simulink model "1DoF_controller_example"  (R2024b)
settings: Solver=FixedStepAuto  StartTime=0.0  StopTime=inf  RelTol=1e-3  EnableMultiTasking=on
undefined symbols (not defined in the file): dspblkCoreblockFVToolHelper, gcbh
libraries: px4Peripheralslib x1, slpidlib x1, px4uORBlib x1, sharedtransform x1, simulink_extras x1
settings Model: SimulationMode=external  ExtModeTrigDuration=10  Creator=luker  LastModifiedBy=luker
settings SolverCC: PositivePriorityOrder=on
settings OptimizationCC: EnhancedBackFolding=on  PassReuseOutputArgsAs=Individual arguments  ZeroExternalMemoryAtStartup=off  ZeroInternalMemoryAtStartup=off  MaxStackSize=64  OptimizeBlockOrder=speed  DifferentSizesBufferReuse=on  EfficientTunableParamExpr=on
settings DebuggingCC: ParameterTunabilityLossMsg=error
settings HardwareCC: ProdBitPerPointer=32  ProdBitPerSizeT=32  ProdBitPerPtrDiffT=32  ProdLargestAtomicInteger=Long  ProdLargestAtomicFloat=Double  ProdWordSize=32  ProdLongLongMode=on  ProdHWDeviceType=ARM Compatible->ARM Cortex
settings SFSimCC: MATLABDynamicMemAlloc=off  SimTargetLang=C++
settings RTWCC: Description=Embedded Coder  SystemTargetFile=ert.tlc  HardwareBoard=PX4 Pixhawk Series  TLCOptions="-aInlineSetEventsForThisBaseRateFcn=TLC_FALSE -aSuppressMultiTaskScheduler=TLC_FALSE  -aRateBasedStepFcn=0"  TemplateMakefile=ert_default_tmf  Toolchain=GNU Tools for PX4 Autopilots  TargetLang=C++
settings CodeAppCC: ForceParamTrailComments=on  IgnoreCustomStorageClasses=off  OperatorAnnotations=on  SimulinkDataObjDesc=on  SFDataObjDesc=on  InsertBlockDesc=on
settings ERTTargetCC: ExtModeTransport=3  ExtModeStaticAlloc=on  ExtModeStaticAllocSize=1024  ExtModeMexFile=ext_xcp  ExtModeIntrfLevel=Level2 - Open  InlinedParameterPlacement=Hierarchical

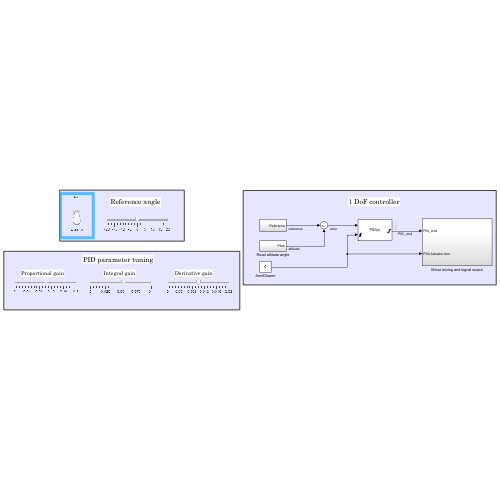
[thumbnail: Simulink's stored preview of the top-level diagram]
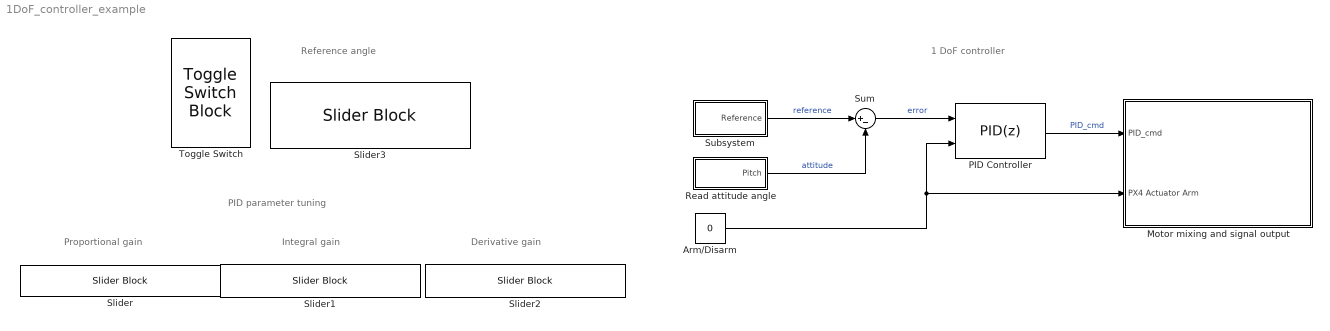
== system 1DoF_controller_example ==
  note: Proportional gain
  note: Reference angle
  note: PID parameter tuning
  note: Integral gain
  note: Derivative gain
  note: 1 DoF controller
  Arm/Disarm : Constant  Value=0
  Motor mixing and signal output : Subsystem
  PID Controller : slpidlib/PID Controller  Controller=PID  Form=Parallel  TimeDomain=Discrete-time  UseExternalTs=off  SampleTime=0.007  IntegratorMethod=Forward Euler  FilterMethod=Forward Euler  ControllerParametersSource=internal  P=0.1027863777089783  I=0.05424823410696267  UseKiTs=off  D=0.01003095975232198  UseExternalDerivativeSource=off  N=60  UseFilter=on  TunerSelectOption=Transfer Function Based (PID Tuner App)  InitialConditionSource=internal  InitialConditionForIntegrator=0  InitialConditionForFilter=0  DifferentiatorICPrevScaledInput=0  ExternalReset=rising  TrackingMode=off  Kt=1  LimitOutput=on  SatLimitsSource=internal  UpperSaturationLimit=0.5  LowerSaturationLimit=-0.5  LinearizeAsGain=off  AntiWindupMode=back-calculation  Kb=100  LimitIntegrator=on  UpperIntegratorSaturationLimit=0.08  LowerIntegratorSaturationLimit=-0.08  POutMin=[]  POutMax=[]  IOutMin=[]  IOutMax=[]  DOutMin=[]  DOutMax=[]  NOutMin=[]  NOutMax=[]  SumOutMin=[]  SumOutMax=[]  SaturationOutMin=[]  SaturationOutMax=[]  PParamMin=[]  PParamMax=[]  IParamMin=[]  IParamMax=[]  DParamMin=[]  DParamMax=[]  NParamMin=[]  NParamMax=[]  KbParamMin=[]  KbParamMax=[]  KtParamMin=[]  KtParamMax=[]  KbOutMin=[]  KbOutMax=[]  KtOutMin=[]  KtOutMax=[]  IntegratorOutMin=[]  IntegratorOutMax=[]  FilterOutMin=[]  FilterOutMax=[]  SumI1OutMin=[]  SumI1OutMax=[]  SumI2OutMin=[]  SumI2OutMax=[]  SumI3OutMin=[]  SumI3OutMax=[]  SumI4OutMin=[]  SumI4OutMax=[]  SumDOutMin=[]  SumDOutMax=[]  DifferentiatorOutMin=[]  DifferentiatorOutMax=[]  FilterDiffOutCoefMin=[]  FilterDiffOutCoefMax=[]  ReciprocalOutMin=[]  ReciprocalOutMax=[]  SumDenOutMin=[]  SumDenOutMax=[]  SumNumOutMin=[]  SumNumOutMax=[]  DivideOutMin=[]  DivideOutMax=[]  UdiffTsProdOutMin=[]  UdiffTsProdOutMax=[]  NTsProdOutMin=[]  NTsProdOutMax=[]  UintegralTsProdOutMin=[]  UintegralTsProdOutMax=[]  UngainTsProdOutMin=[]  UngainTsProdOutMax=[]  ClampingZeroOutDataTypeStr=Inherit: Inherit via back propagation  ClampingZeroOutMin=[]  ClampingZeroOutMax=[]  FilterDenConstantOutDataTypeStr=Inherit: Inherit via back propagation  FilterDenConstantOutMin=[]  FilterDenConstantOutMax=[]  PCopyOutDataTypeStr=Inherit: Inherit via back propagation  PCopyOutMin=[]  PCopyOutMax=[]  NCopyOutDataTypeStr=Inherit: Inherit via back propagation  NCopyOutMin=[]  NCopyOutMax=[]  IntegratorContinuousStateAttributes=''  IntegratorStateMustResolveToSignalObject=off  IntegratorRTWStateStorageClass=Auto  FilterContinuousStateAttributes=''  FilterStateMustResolveToSignalObject=off  FilterRTWStateStorageClass=Auto  ParallelPVariant=InternalParameters  IdealPVariant=Disabled  IVariant=InternalParameters  DVariant=InternalParameters  IntegratorVariant=Discrete  SatVariant=Enabled  AWVariant=BackCalculation  PCopyVariant=Disabled  TRVariant=Disabled  FdbkBlocksVariant=Forward  IdealPFdbkVariant=Disabled  SatFdbkVariant=Disabled  DerivativeFilterVariant=ForwardEulerFilter  NVariant=InternalParameters  NCopyVariant=Disabled  FilterICVariant=InternalICsFilter  IntegratorICVariant=InternalICs  ExternalResetVariant=ExternalReset  TRSumVariant=Passthrough  SumFdbkVariant=Disabled  SumVariant=Sum_PID  TsampFilterVariant=InternalTs  TsampNgainVariant=Passthrough  TsampIntegralVariant=Disabled_SignalSpec  ExternalSaturationOutDataTypeStr=Inherit: Same as second input  DerivativeSourceVariant=ErrorSignal  PreIntVariant=InternalPreInt
  Read attitude angle : Subsystem
  Slider : SliderBlock  LabelPosition=Hide  ScaleMax=0.2
  Slider1 : SliderBlock  LabelPosition=Hide  ScaleMax=0.1
  Slider2 : SliderBlock  LabelPosition=Hide  ScaleMax=0.02
  Slider3 : SliderBlock  LabelPosition=Hide  ScaleMin=-20  ScaleMax=20  TickInterval=5
  Subsystem : Subsystem
  Sum : Sum  Inputs=|+-
  Toggle Switch : ToggleSwitchBlock  LabelPosition=Hide
      settings: Values={{'Disarm', 'Arm'}, [0 1]}
  wires:
  Arm/Disarm/1 -> PID Controller/2, Motor mixing and signal output/2(PX4 Actuator Arm)
  Subsystem/1(Reference) -> Sum/1  "reference"
  Read attitude angle/1(Pitch) -> Sum/2  "attitude"
  Sum/1 -> PID Controller/1  "error"
  PID Controller/1 -> Motor mixing and signal output/1(PID_cmd)  "PID_cmd"

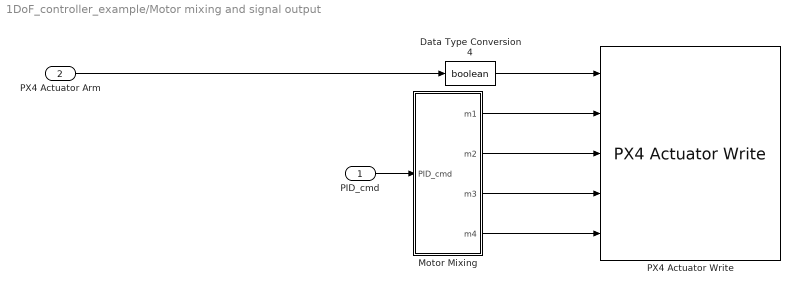
== system 1DoF_controller_example/Motor mixing and signal output ==
  PID_cmd : Inport
  PX4 Actuator Arm : Inport  Port=2
  Data Type Conversion4 : DataTypeConversion  OutDataTypeStr=boolean  SaturateOnIntegerOverflow=off  RndMeth=Floor
  Motor Mixing : Subsystem
  PX4 Actuator Write : px4Peripheralslib/PX4 Actuator Write  Motor1Enable=on  Motor2Enable=on  Motor3Enable=on  Motor4Enable=on  Motor5Enable=off  Motor6Enable=off  Motor7Enable=off  Motor8Enable=off  Motor9Enable=off  Motor10Enable=off  Motor11Enable=off  Motor12Enable=off  IsMotorArray=off  Servo1Enable=off  Servo2Enable=off  Servo3Enable=off  Servo4Enable=off  Servo5Enable=off  Servo6Enable=off  Servo7Enable=off  Servo8Enable=off  IsServoArray=off
  wires:
  Motor Mixing/2(m2) -> PX4 Actuator Write/3
  Data Type Conversion4/1 -> PX4 Actuator Write/1
  PID_cmd/1 -> Motor Mixing/1(PID_cmd)
  Motor Mixing/3(m3) -> PX4 Actuator Write/4
  Motor Mixing/1(m1) -> PX4 Actuator Write/2
  PX4 Actuator Arm/1 -> Data Type Conversion4/1
  Motor Mixing/4(m4) -> PX4 Actuator Write/5

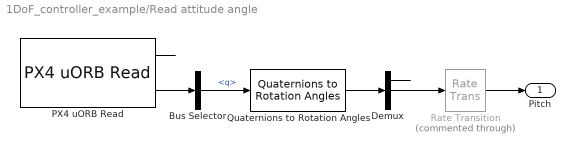
== system 1DoF_controller_example/Read attitude angle ==
  Bus Selector : BusSelector  OutputSignals=q
  Demux : Demux  Outputs=3
  PX4 uORB Read : px4uORBlib/PX4 uORB Read  uORBTopic=VehicleAttitude  selectInstance=vehicle_attitude  SampleTime=-1  BlockingMode=off  BlockTimeout=1e-3
  Quaternions to Rotation Angles : sharedtransform/Quaternions to Rotation Angles  rotationOrder=ZYX  aMode=aMode
  Rate Transition : RateTransition  Commented=through  OutPortSampleTime=0.007
  Pitch : Outport
  wires:
  PX4 uORB Read/1 -> ?
  PX4 uORB Read/2 -> Bus Selector/1
  Quaternions to Rotation Angles/1 -> Demux/1
  Demux/1 -> ?
  Demux/2 -> Rate Transition/1
  Bus Selector/1 -> Quaternions to Rotation Angles/1  "<q>"
  Rate Transition/1 -> Pitch/1

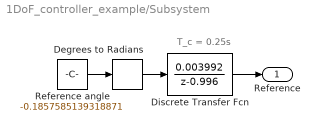
== system 1DoF_controller_example/Subsystem ==
  note: T_c = 0.25s
  Degrees to Radians : simulink_extras/Transformations/Degrees to Radians
  Discrete Transfer Fcn : DiscreteTransferFcn  LoadFcn=dspblkCoreblockFVToolHelper(gcbh,'load');  Numerator=[0.003992]  Denominator=[1 -0.996]
      settings: CopyFcn=dspblkCoreblockFVToolHelper(gcbh,'copy');  DeleteFcn=dspblkCoreblockFVToolHelper(gcbh,'close');  ModelCloseFcn=dspblkCoreblockFVToolHelper(gcbh,'close');  PreSaveFcn=dspblkCoreblockFVToolHelper(gcbh,'presave');  PostSaveFcn=dspblkCoreblockFVToolHelper(gcbh,'postsave');  CloseFcn=dspblkCoreblockFVToolHelper(gcbh,'close');
  Reference angle : Constant  Value=-0.1857585139318871
  Reference : Outport
  wires:
  Reference angle/1 -> Degrees to Radians/1
  Degrees to Radians/1 -> Discrete Transfer Fcn/1
  Discrete Transfer Fcn/1 -> Reference/1

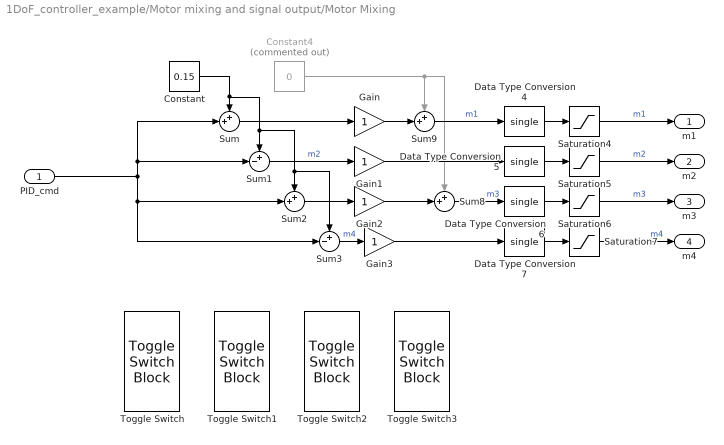
== system 1DoF_controller_example/Motor mixing and signal output/Motor Mixing ==
  PID_cmd : Inport
  Constant : Constant  Value=0.15
  Constant4 : Constant  Commented=on  Value=0
  Data Type Conversion{4..7} (4 alike) : DataTypeConversion  OutDataTypeStr=single  SaturateOnIntegerOverflow=off  RndMeth=Floor
  Gain{,1..3} (4 alike) : Gain
  Saturation{4..7} (4 alike) : Saturate  UpperLimit=1  LowerLimit=0
  Sum{,2,8..9} (4 alike) : Sum  Inputs=++|
  Sum1 : Sum  Inputs=+-|
  Sum3 : Sum  Inputs=+-|
  Toggle Switch{,1..3} (4 alike) : ToggleSwitchBlock
      settings: Values={{'Off', 'On'}, [0 1]}
  m1 : Outport
  m2 : Outport  Port=2
  m3 : Outport  Port=3
  m4 : Outport  Port=4
  wires:
  Constant/1 -> Sum1/1, Sum3/1, Sum2/1, Sum/1
  Sum2/1 -> Gain2/1
  Constant4/1 -> Sum9/1, Sum8/1
  Sum/1 -> Gain/1
  Sum9/1 -> Data Type Conversion4/1  "m1"
  Sum8/1 -> Data Type Conversion6/1  "m3"
  Sum3/1 -> Gain3/1  "m4"
  Sum1/1 -> Gain1/1  "m2"
  Saturation4/1 -> m1/1  "m1"
  Saturation5/1 -> m2/1  "m2"
  Saturation6/1 -> m3/1  "m3"
  Saturation7/1 -> m4/1  "m4"
  Data Type Conversion4/1 -> Saturation4/1
  Data Type Conversion5/1 -> Saturation5/1
  Data Type Conversion6/1 -> Saturation6/1
  Data Type Conversion7/1 -> Saturation7/1
  Gain/1 -> Sum9/2
  Gain1/1 -> Data Type Conversion5/1
  Gain2/1 -> Sum8/2
  Gain3/1 -> Data Type Conversion7/1
  PID_cmd/1 -> Sum2/2, Sum3/2, Sum1/2, Sum/2
